simulink model "Simulation1"  (R2024a)
settings: Solver=ode3  StartTime=0.0  StopTime=inf  FixedStep=0.002  RelTol=1e-3  EnableMultiTasking=on
libraries: quarc_library x2
settings Model: ExtModeTrigDuration=10000  Creator=schuster.t  LastModifiedBy=schuster.t
settings SolverCC: AlgebraicLoopSolver=TrustRegion  PositivePriorityOrder=on
settings DataIOCC: ReturnWorkspaceOutputs=off
settings DebuggingCC: UnconnectedInputMsg=warning  UnconnectedOutputMsg=warning  UnconnectedLineMsg=warning  ArithmeticOperatorsInVariantConditions=warning
settings ModelReferenceCC: EnableRefExpFcnMdlSchedulingChecks=on
settings SFSimCC: SimUseLocalCustomCode=off  CustomCodeUndefinedFunction=UseInterfaceOnly
settings RTWCC: Description=QUARC Win64 Target Using Toolchain  SystemTargetFile=quarc_win64.tlc  TemplateMakefile=quarc_default_tmf  RTWUseLocalCustomCode=off  Toolchain=QUARC win64 | nmake (64-bit Windows)  BuildConfiguration=Faster Runs  GPUComputeCapability=3.5
settings CodeAppCC: StateflowObjectComments=on
settings STFCustomTargetCC: ConcurrentExecutionCompliant=on  SystemTargetFile=quarc_win64.tlc
settings GRTTargetCC: ParMdlRefBuildCompliant=off  CompOptLevelCompliant=off  CombineOutputUpdateFcns=off  MatFileLogging=off  CPPClassGenCompliant=off  GRTInterface=on  ExtMode=on  ExtModeMexFile=quarc_comm
settings ConfigComp: CovMetricSettings=dswe

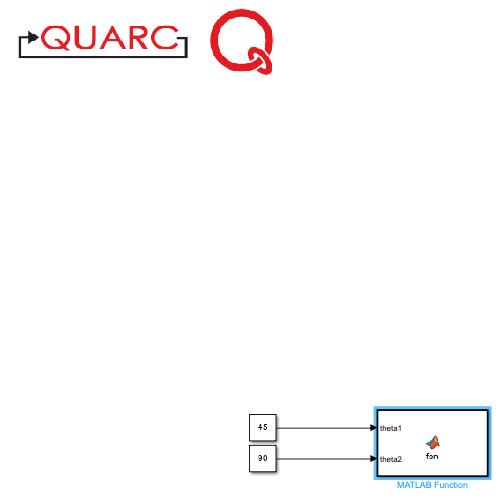
[thumbnail: Simulink's stored preview of the top-level diagram]
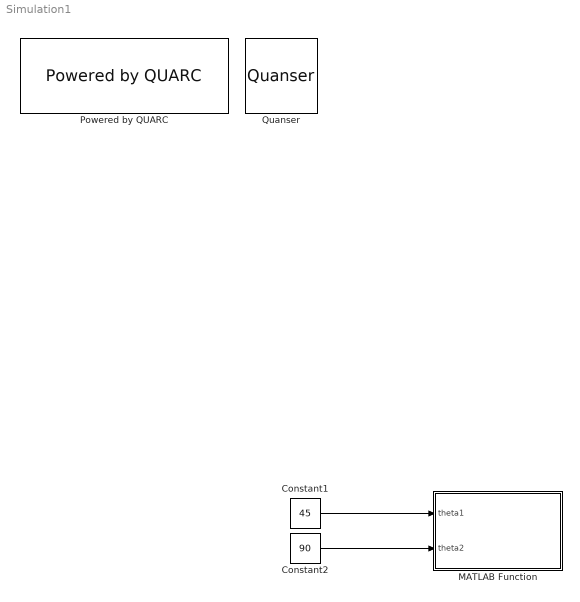
== system Simulation1 ==
  Constant1 : Constant  Value=45
  Constant2 : Constant  Value=90
  MATLAB Function : MATLAB Function  TreatAsAtomicUnit=on
  Powered by QUARC : quarc_library/Logos/Powered by QUARC
  Quanser : quarc_library/Logos/Quanser
  wires:
  Constant2/1 -> MATLAB Function/2(theta2)
  Constant1/1 -> MATLAB Function/1(theta1)

== matlab function Simulation1/MATLAB Function ==
  data: theta1 input; theta2 input
function fcn(theta1, theta2)
    BaseDesX = [0, 0];
    BaseDesY = [0, 0];
    BaseDesZ = [-5, 0];
    plot3(BaseDesX,BaseDesY,BaseDesZ,'rs-', 'LineWidth', 2, 'MarkerSize', 8);     
    hold on
    grid on
    axis([-20 20 -20 20 -5 15])
    points1 = [0 0 0 1; 0 0 -1 1; 0 6 -1 1; 0 6 0 1; 0 8 0 1]';
    [transformedLink1, transformedMatrix1] = TRANS0_1(theta1, points1);
    link2points = [0 0 0 1; 0 12 0 1]';
    link2transf = TRANS1_2(theta2, 8, link2points, transformedMatrix1);
    plot3(link2transf(1,:), link2transf(2,:), link2transf(3,:), 'b-');
    plot3(transformedMatrix1(1,:), transformedMatrix1(2,:), transformedMatrix1(3,:), 'ro-');
end
